simulink model "PSM2_Gruppe7B_Testumgebung"  (R2012b)
settings: Solver=FixedStepDiscrete  StartTime=0.0  StopTime=1  RelTol=1e-3
libraries: idelinklib_tgtpref x1
settings Model: Creator=Nikolay  LastModifiedBy=Nikolay
settings DataIOCC: SaveOutput=off  SaveTime=off
settings OptimizationCC: OptimizeModelRefInitCode=on  LifeSpan=1
settings HardwareCC: ProdBitPerChar=16  ProdBitPerInt=16  ProdBitPerPointer=16  ProdLargestAtomicInteger=Integer  ProdIntDivRoundTo=Zero  ProdEndianess=LittleEndian  ProdWordSize=16  ProdHWDeviceType=Texas Instruments->C2000
settings RTWCC: SystemTargetFile=idelink_ert.tlc  GenerateMakefile=off  TemplateMakefile=none  Description=IDE Link ERT  ProcessScript=idelink_ert_make_rtw_hook
settings CodeAppCC: IgnoreCustomStorageClasses=off

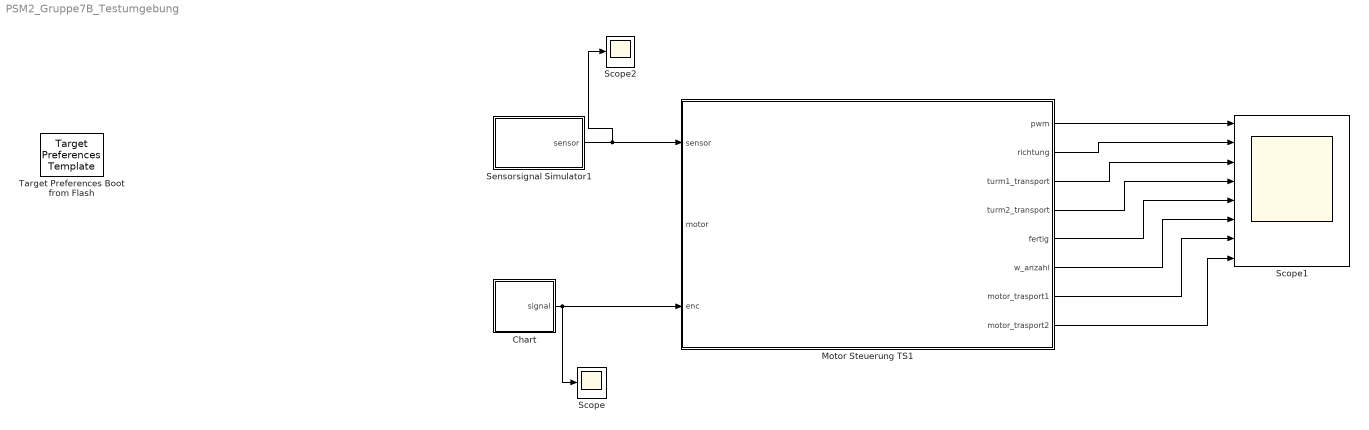
== system PSM2_Gruppe7B_Testumgebung ==
  Chart : Stateflow chart  TreatAsAtomicUnit=on
  Motor Steuerung TS1 : Stateflow chart  TreatAsAtomicUnit=on
  Scope : Scope
  Scope1 : Scope  NumInputPorts=8
      settings: YMin=-5~-5~-5~-5~-5~-5~-5~-5  YMax=5~5~5~5~5~5~5~5
  Scope2 : Scope
      settings: SaveName=ScopeData2
  Sensorsignal Simulator1 : Stateflow chart  TreatAsAtomicUnit=on
  Target Preferences Boot from Flash : idelinklib_tgtpref/Target Preferences Template  Tag=ccslinktgtpref_ccsv4  library=off
  wires:
  Chart/1(signal) -> Motor Steuerung TS1/3(enc), Scope/1
  Sensorsignal Simulator1/1(sensor) -> Scope2/1, Motor Steuerung TS1/1(sensor)
  Motor Steuerung TS1/1(pwm) -> Scope1/1
  Motor Steuerung TS1/2(richtung) -> Scope1/2
  Motor Steuerung TS1/3(turm1_transport) -> Scope1/3
  Motor Steuerung TS1/4(turm2_transport) -> Scope1/4
  Motor Steuerung TS1/5(fertig) -> Scope1/5
  Motor Steuerung TS1/6(w_anzahl) -> Scope1/6
  Motor Steuerung TS1/7(motor_trasport1) -> Scope1/7
  Motor Steuerung TS1/8(motor_trasport2) -> Scope1/8

== stateflow chart PSM2_Gruppe7B_Testumgebung/Motor Steuerung TS1 ==
  state Sensor_handler [parallel]
    settings: executionOrder=5
    state Start
      ex: s_counter = 0
    state Check_sensor
    state Wuerfel_kommt
    state Anzahl_berechnen
      anz = s_counter/1;
    state Wuerfel_incrementieren
      w_anzahl = w_anzahl + anz;
    (default) -> Sensor_handler.Start
    Wuerfel_incrementieren -> Sensor_handler.Start
    Sensor_handler.Start -> Check_sensor
    Wuerfel_kommt -> Check_sensor : {s_counter++}
    Check_sensor -> Wuerfel_kommt [order 2] : [sensor == 0]
    Check_sensor -> Anzahl_berechnen [order 1] : [sensor == 1]
    Anzahl_berechnen -> Wuerfel_incrementieren
  state Motor_Foerderbahn_Check [parallel]
    settings: executionOrder=3
    state Start
    state Encoder_abfrage
      zustand_vor = enc;
    state Naechster_Wert
      zustand_nach = enc;
    state Vergleich
      vrgl = zustand_nach - zustand_vor;
    state Nicht_Verklemmt
      verklemmung = false;
    state Verklemmt
      verklemmung = true;
    Nicht_Verklemmt -> Motor_Foerderbahn_Check.Start
    Verklemmt -> Motor_Foerderbahn_Check.Start
    Motor_Foerderbahn_Check.Start -> Encoder_abfrage : [TS2_aktiv == false & TS3_aktiv == false]
    Encoder_abfrage -> Naechster_Wert : [after(3,tick)]
    Naechster_Wert -> Vergleich
    Vergleich -> Nicht_Verklemmt [order 1] : [abs(vrgl) == 1]
    Vergleich -> Verklemmt [order 2] : [abs(vrgl) == 0]
  state Teilsystem_2 [parallel]
    settings: executionOrder=6
    state Start
    state TS1_stop
      TS2_aktiv = true;
    state Platforme_hoch_1
      PM_richtung = 0;
      PM_pwm = 60;
    state Stab_entfernen
      WM_pwm = 0;
      SM_richtung = 0;
      SM_pwm = 60;
    state Platforme_hoch_2
      SM_pwm = 0;
      PM_pwm = 60;
    state Stab_setzen
    (default) -> Teilsystem_2.Start
    Teilsystem_2.Start -> Teilsystem_2.TS1_stop : [sensor == 0]
    Teilsystem_2.TS1_stop -> Platforme_hoch_1
    Platforme_hoch_1 -> Stab_entfernen : after(25000,tick)
    Stab_entfernen -> Platforme_hoch_2 : after(25000,tick)
    Platforme_hoch_2 -> Stab_setzen : []
  state Verklemmung_entfernen [parallel]
    settings: executionOrder=4
    state Start
      FM_pwm = 60;
      richtung = 0
    state Motor_rueckwaerts
      FM_richtung = 1;
      FM_pwm = 80;
    state Check_wieder
    (default) -> Verklemmung_entfernen.Start
    Check_wieder -> Verklemmung_entfernen.Start [order 2]
    Verklemmung_entfernen.Start -> Motor_rueckwaerts : [verklemmung == true && TS3_aktiv == false]
    Check_wieder -> Motor_rueckwaerts [order 1] : [verklemmung == true]
    Motor_rueckwaerts -> Check_wieder : after(5,tick)
  state Teilsystem_1 [parallel]
    settings: executionOrder=1
    state Start
      en: FM_pwm = 60;
      FM_richtung = 0;
      w_anzahl = 0;
    state Abfrage_Wuerfel
      en: turm_checker();
    state System_idle
      FM_pwm = 0;
    (default) -> Teilsystem_1.Start
    Teilsystem_1.System_idle -> Teilsystem_1.Start : [TS3_aktiv == false && TS2_aktiv = false ]
    Teilsystem_1.Start -> Abfrage_Wuerfel
    Abfrage_Wuerfel -> Teilsystem_1.System_idle [order 2] : [TS3_aktiv == true || TS2_aktiv == true]
    Abfrage_Wuerfel -> Abfrage_Wuerfel [order 1] : [TS3_aktiv == false]
  state Teilsystem_3 [parallel]
    settings: executionOrder=2
    state Start
    state System_idle
      TS3_aktive = false;
    state TS1_stop
      TS3_aktiv = true;
    state Drehen_zureuck
      SM_pwm = 0;
      DM_richtung = 1;
      DM_PWM = 60;
    state Magazin_transport
      TM1_richtung = 0;
      TM2_richtung = 0;
      TM1_PWM = 100;
      TM2_PWM = 100;
    state Schieber_zureuck
      SM_richtung = 1;
      SM_pwm = 60;
    state Hohe_abfrage
    state Schieber_warten
      SM_pwm = 0;
    state Drehen_T1
      DM_pwm = 60;
      DM_richtung = 0
      tum1_transport = false;
    state Schieber
      DM_pwm =0
      SM_richtung = 0;
      SM_pwm = 60;
    state Drehen_T2
      DM_pwm = 60;
      DM_richtung = 0
      tum2_transport = false;
    (default) -> Teilsystem_3.Start
    Teilsystem_3.System_idle -> Teilsystem_3.Start
    Teilsystem_3.Start -> Teilsystem_3.TS1_stop : [turm1_transport == true || turm2_transport == true ]
    Drehen_zureuck -> Teilsystem_3.System_idle : [knopf_gedrueckt == true]
    Teilsystem_3.TS1_stop -> Magazin_transport
    Schieber_zureuck -> Drehen_zureuck : after(1,sec)
    Magazin_transport -> Hohe_abfrage
    Schieber_warten -> Schieber_zureuck : after(25000,tick)
    Hohe_abfrage -> (junction 262)
    Schieber -> Schieber_warten : after(1,sec)
    (junction 262) -> Drehen_T1 [order 1] : [turm1_transport == true]
    Drehen_T1 -> Schieber : after(2,sec)
    (junction 262) -> Drehen_T2 [order 2] : turm2_transport == true]
    Drehen_T2 -> Schieber : after(3,sec)
  state turm_checker [function]
    (default) -> (junction 107) : /* turm_checker */
    (junction 107) -> (junction 109) [order 1] : [turm1_gebaut == false && w_anzahl == 6]
    (junction 107) -> (junction 108) [order 2]
    (junction 109) -> (junction 114) : {turm1_transport = true; turm1_gebaut = true; w_anzahl = 0;}
    (junction 108) -> (junction 113) [order 1] : [turm1_gebaut == true && turm2_gebaut == false && w_anzahl == 9]
    (junction 108) -> (junction 115) [order 2]
    (junction 113) -> (junction 110) : {turm1_gebaut = true; turm2_gebaut = true; w_anzahl = 0;}
    (junction 115) -> (junction 116) [order 1] : [turm1_gebaut == true && turm2_gebaut == true]
    (junction 115) -> (junction 111) [order 2] : {fertig = false;}
    (junction 116) -> (junction 117) : {fertig = true;}
    (junction 117) -> (junction 111)
    (junction 110) -> (junction 117)
    (junction 114) -> (junction 110)
    (junction 111) -> (junction 112)
  state r_zahler(T) [function]
    (default) -> (junction 194) : /* Rueckwaert Zaehler */
    (junction 194) -> (junction 191)
    (junction 191) -> (junction 193) [order 1] : [T!=0]
    (junction 193) -> (junction 190) : {T--;}
    (junction 190) -> (junction 191)
    (junction 191) -> (junction 192) [order 2]
  data: T function_input double; sensor input; pwm output double; richtung output double; turm1_transport output double; turm2_transport output double; fertig output double; w_anzahl output double; turm1_gebaut local double; turm2_gebaut local double; motor input; r_zaehl local double; verklemmung local double; vrgl local double; zustand_nach local double; zustand_vor local double; motor_trasport1 output double; motor_trasport2 output double; enc input; TS2_aktiv local double; anz local double; s_counter local double

== stateflow chart PSM2_Gruppe7B_Testumgebung/Chart ==
  state Bip
    signal = 1;
  state Bop
    signal = 0;
  (default) -> Bip
  Bip -> Bop : after(3,tick)
  Bop -> Bip : after(3,tick)
  data: signal output double

== stateflow chart PSM2_Gruppe7B_Testumgebung/Sensorsignal Simulator1 ==
  state Start
    sensor = 1;
  state Sensor_an
    sensor = 0
  (default) -> Start
  Sensor_an -> Start : after(2,tick)
  Start -> Sensor_an : after(1,tick)
  data: sensor output double
